simulink model "VD_correct"  (R2023b)
settings: Solver=ode113  StartTime=0.0  StopTime=20  MaxStep=0.4  RelTol=1e-3
libraries: simulink x2, slpidlib x1
settings Model: Creator=Supriya  LastModifiedBy=Supriya

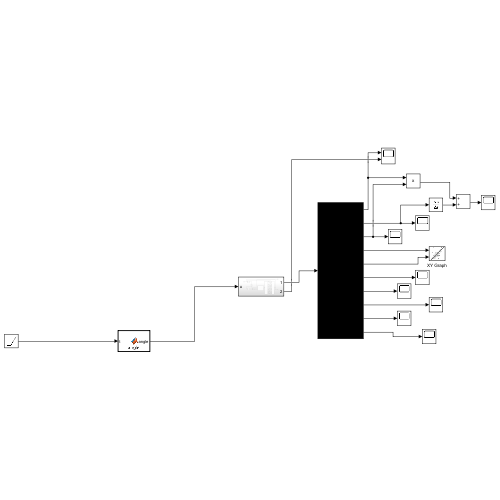
[thumbnail: Simulink's stored preview of the top-level diagram]
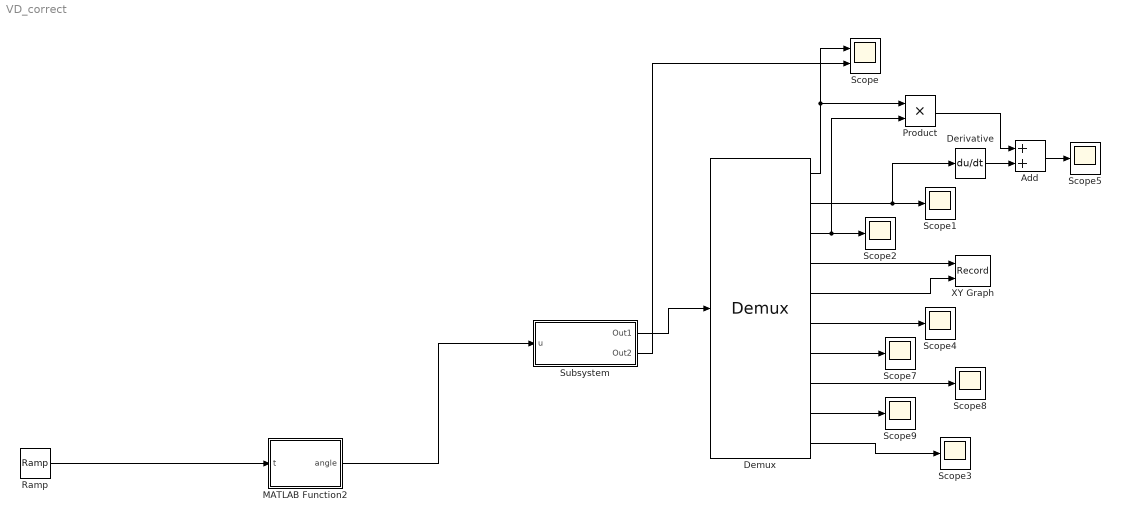
== system VD_correct ==
  Add : Sum
  Demux : Demux  Outputs=10
  Derivative : Derivative
  MATLAB Function2 : MATLAB Function  TreatAsAtomicUnit=on
  Product : Product
  Ramp : simulink/Sources/Ramp  slope=1  start=0  InitialOutput=0
  Scope : Scope  NumInputPorts=2
  Scope{1..5,7..9} (8 alike) : Scope
  Subsystem : Subsystem
  XY Graph : Record  FileSettingsInternal="{\"entries\":[{\"content\":{\"excelSettings\":{\"content\":{},\"type\":\"Streamout.ExcelSettings\"}},\"type\":\"Streamout.FileSettingStorage\",\"uuid\":\"\"}],\"packageUris\":[\"http:\\/\\/schema.mathworks.com\\/mf0\\/streamout_blocks\\/R2020a\"],\"version\":\"1.0\"}"  Layout=[1 1]  SignalsInternal="{\"entries\":[{\"content\":{\"signals\":[{\"content\":{\"blockPath\":[],\"dimensions\":[1],\"domain\":\"\",\"lineColor\":\"#a2142f\",\"plots\":[ 1 ],\"port\":1,\"sid\":[\"\"],\"signalID\":1,\"signalName\":\"Demux:4\"},\"type\":\"RecordBlkView.Signal\",\"uuid\":\"\"},{\"content\":{\"blockPath\":[],\"dimensions\":[1],\"domain\":\"\",\"lineColor\":\"#139fff\",\"plots\":[ 1 ],\"port\":2,\"sid\":[\"\"],\"signalID\":2,\"signalName\":\"Demux:5\"},\"type\":\"RecordBlkView.Signal\",\"uuid\":\"\"}]},\"type\":\"RecordBlkView.InputSignals\",\"uuid\":\"\"}],\"packageUris\":[\"http:\\/\\/schema.mathworks.com\\/mf0\\/streamout_blocks\\/R2020a\"],\"version\":\"1.0\"}"  VisualizationBindings="{\"xyplotplugin\":{\"info\":[{\"series\":[{\"bindingParametersList\":[{\"parameter\":\"X-Axis\",\"signalID\":1,\"signalName\":\"Demux:4\"},{\"parameter\":\"Y-Axis\",\"signalID\":2,\"signalName\":\"Demux:5\"}],\"seriesID\":0}],\"subplotID\":1}]}}"  CompatibilityTag=XY
  wires:
  Ramp/1 -> MATLAB Function2/1(t)
  MATLAB Function2/1(angle) -> Subsystem/1(u)
  Subsystem/1(Out1) -> Demux/1
  Demux/1 -> Scope/1, Product/1
  Demux/2 -> Derivative/1, Scope1/1
  Demux/3 -> Product/2, Scope2/1
  Demux/6 -> Scope4/1
  Demux/4 -> XY Graph/1
  Demux/5 -> XY Graph/2
  Demux/7 -> Scope7/1
  Demux/8 -> Scope8/1
  Demux/9 -> Scope9/1
  Demux/10 -> Scope3/1
  Product/1 -> Add/1
  Derivative/1 -> Add/2
  Add/1 -> Scope5/1
  Subsystem/2(Out2) -> Scope/2

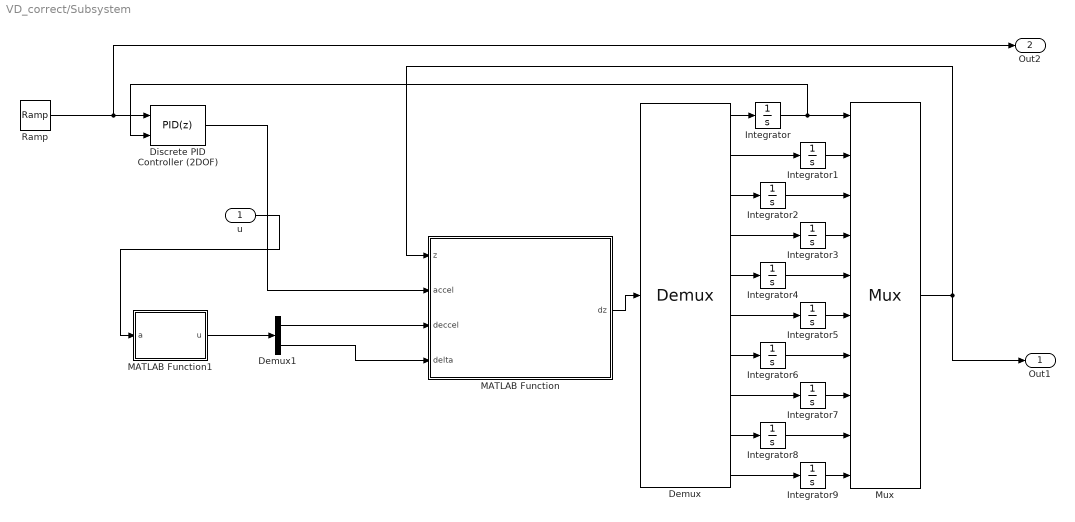
== system VD_correct/Subsystem ==
  u : Inport
  Demux : Demux  Outputs=10
  Demux1 : Demux  Outputs=2
  Discrete PID Controller (2DOF) : slpidlib/PID Controller (2DOF)  Controller=PID  Form=Parallel  TimeDomain=Discrete-time  UseExternalTs=off  SampleTime=-1  IntegratorMethod=Forward Euler  FilterMethod=Forward Euler  ControllerParametersSource=internal  P=6.4  I=8  UseKiTs=off  D=0.4  N=100  UseFilter=off  b=1  c=1  TunerSelectOption=Transfer Function Based (PID Tuner App)  InitialConditionSource=internal  InitialConditionForIntegrator=0  InitialConditionForFilter=0  DifferentiatorICPrevScaledInput=0  ExternalReset=none  TrackingMode=off  Kt=1  LimitOutput=off  SatLimitsSource=internal  UpperSaturationLimit=inf  LowerSaturationLimit=-inf  LinearizeAsGain=off  AntiWindupMode=none  Kb=1  LimitIntegrator=off  UpperIntegratorSaturationLimit=inf  LowerIntegratorSaturationLimit=-inf  POutMin=[]  POutMax=[]  IOutMin=[]  IOutMax=[]  DOutMin=[]  DOutMax=[]  NOutMin=[]  NOutMax=[]  bOutMin=[]  bOutMax=[]  cOutMin=[]  cOutMax=[]  SumOutMin=[]  SumOutMax=[]  SaturationOutMin=[]  SaturationOutMax=[]  PParamMin=[]  PParamMax=[]  IParamMin=[]  IParamMax=[]  DParamMin=[]  DParamMax=[]  NParamMin=[]  NParamMax=[]  bParamMin=[]  bParamMax=[]  cParamMin=[]  cParamMax=[]  KbParamMin=[]  KbParamMax=[]  KtParamMin=[]  KtParamMax=[]  KbOutMin=[]  KbOutMax=[]  KtOutMin=[]  KtOutMax=[]  IntegratorOutMin=[]  IntegratorOutMax=[]  FilterOutMin=[]  FilterOutMax=[]  SumI1OutMin=[]  SumI1OutMax=[]  SumI2OutMin=[]  SumI2OutMax=[]  SumI3OutMin=[]  SumI3OutMax=[]  SumI4OutMin=[]  SumI4OutMax=[]  SumDOutMin=[]  SumDOutMax=[]  Sum1OutMin=[]  Sum1OutMax=[]  Sum2OutMin=[]  Sum2OutMax=[]  Sum3OutMin=[]  Sum3OutMax=[]  DifferentiatorOutMin=[]  DifferentiatorOutMax=[]  FilterDiffOutCoefMin=[]  FilterDiffOutCoefMax=[]  ReciprocalOutMin=[]  ReciprocalOutMax=[]  SumDenOutMin=[]  SumDenOutMax=[]  SumNumOutMin=[]  SumNumOutMax=[]  DivideOutMin=[]  DivideOutMax=[]  UdiffTsProdOutMin=[]  UdiffTsProdOutMax=[]  NTsProdOutMin=[]  NTsProdOutMax=[]  UintegralTsProdOutMin=[]  UintegralTsProdOutMax=[]  UngainTsProdOutMin=[]  UngainTsProdOutMax=[]  ClampingZeroOutDataTypeStr=Inherit: Inherit via back propagation  ClampingZeroOutMin=[]  ClampingZeroOutMax=[]  FilterDenConstantOutDataTypeStr=Inherit: Inherit via back propagation  FilterDenConstantOutMin=[]  FilterDenConstantOutMax=[]  PCopyOutDataTypeStr=Inherit: Inherit via back propagation  PCopyOutMin=[]  PCopyOutMax=[]  NCopyOutDataTypeStr=Inherit: Inherit via back propagation  NCopyOutMin=[]  NCopyOutMax=[]  IntegratorContinuousStateAttributes=''  IntegratorStateMustResolveToSignalObject=off  IntegratorRTWStateStorageClass=Auto  FilterContinuousStateAttributes=''  FilterStateMustResolveToSignalObject=off  FilterRTWStateStorageClass=Auto  ParallelPVariant=InternalParameters  IdealPVariant=Disabled  IVariant=InternalParameters  DVariant=InternalParameters  bVariant=InternalParameters  cVariant=InternalParameters  IntegratorVariant=Discrete  SatVariant=Disabled  AWVariant=Passthrough  PCopyVariant=Disabled  TRVariant=Disabled  FdbkBlocksVariant=Forward  IdealPFdbkVariant=Disabled  SatFdbkVariant=Disabled  DerivativeFilterVariant=Differentiator  NVariant=Passthrough  NCopyVariant=Disabled_SignalSpec  FilterICVariant=InternalICsDifferentiator  IntegratorICVariant=InternalICs  ExternalResetVariant=Disabled  TRSumVariant=Passthrough  SumFdbkVariant=Disabled  SumVariant=Sum_PID  TsampFilterVariant=InternalTs  TsampNgainVariant=Passthrough  TsampIntegralVariant=Disabled_SignalSpec  ExternalSaturationOutDataTypeStr=Inherit: Same as second input
      settings: LibrarySourceBlock=simulink/Discrete/Discrete PID Controller (2DOF)
  Integrator : Integrator  InitialCondition=16
  Integrator{1..9} (9 alike) : Integrator
  MATLAB Function : MATLAB Function  TreatAsAtomicUnit=on
  MATLAB Function1 : MATLAB Function  TreatAsAtomicUnit=on
  Mux : Mux  Inputs=10
  Ramp : simulink/Sources/Ramp  slope=0.64  start=0  InitialOutput=16
  Out1 : Outport
  Out2 : Outport  Port=2
  wires:
  MATLAB Function/1(dz) -> Demux/1
  Demux/1 -> Integrator/1
  Integrator/1 -> Discrete PID Controller (2DOF)/2, Mux/1
  Demux/3 -> Integrator2/1
  Integrator2/1 -> Mux/3
  Integrator1/1 -> Mux/2
  Demux/2 -> Integrator1/1
  Demux/4 -> Integrator3/1
  Integrator3/1 -> Mux/4
  Integrator4/1 -> Mux/5
  Demux/5 -> Integrator4/1
  Demux/6 -> Integrator5/1
  Integrator5/1 -> Mux/6
  Demux/7 -> Integrator6/1
  Integrator6/1 -> Mux/7
  Demux/8 -> Integrator7/1
  Integrator7/1 -> Mux/8
  Demux/9 -> Integrator8/1
  Integrator8/1 -> Mux/9
  Demux/10 -> Integrator9/1
  Integrator9/1 -> Mux/10
  Mux/1 -> MATLAB Function/1(z), Out1/1
  u/1 -> MATLAB Function1/1(a)
  MATLAB Function1/1(u) -> Demux1/1
  Discrete PID Controller (2DOF)/1 -> MATLAB Function/2(accel)
  Ramp/1 -> Out2/1, Discrete PID Controller (2DOF)/1
  Demux1/1 -> MATLAB Function/3(deccel)
  Demux1/2 -> MATLAB Function/4(delta)

== matlab function VD_correct/Subsystem/MATLAB Function1 ==
  data: a input; u output
function u = u(a)
    u=[0, a];
end

== matlab function VD_correct/MATLAB Function2 ==
  data: t input; angle output
function angle = angle(t)
    % if t<1
    %     angle_steer = 0;%(pi/180) * sin(2*pi*0.1*t);
    % elseif 16>=t>=1
    %     angle_steer = 0.5*(pi/180)*t;
    % else
    %     angle_steer=8*(pi/180)*t;
    % end
    angle_steer = 3*(pi/180) * sin(2*pi*0.2*t);
    angle=angle_steer;
end

== matlab function VD_correct/Subsystem/MATLAB Function ==
  data: dz output; z input; accel input; deccel input; delta input
%This code is for state space of vehicle dynamics
% states: Vx, Vy, r

function dz = vehicle_dynamics(z, accel,deccel,delta)
    % abc = Forces
    % dt;
    %tic;    
    dz =zeros(10,1);
    params = system_parameters();
    Vx =  z(1);
    Vy = z(2);
    r  = z(3);
    x  = z(4);
    y  = z(5);
    psi= z(6);
    ax = -z(2) * r;
    ay = z(1) * r;

    %%input torue to each wheel 
    tau_in = cal_wheel_torque_in(params, accel, deccel);
    tau_in_fl = tau_in(1);
    tau_in_fr = tau_in(2);
    tau_in_rl = tau_in(3);
    tau_in_rr = tau_in(4);
    
    %% calculate forces
    t_forces = tire_forces(params, z, delta, ax, ay, deccel); %8 * 1 vector
    [Fx_sum, Fy_f, Fy_r, Fy_del] = vehicle_forces(params, z, t_forces, delta);
        
    Vx_dt = Vy * r + (Fx_sum / params.m);
    Vy_dt = -Vx * r + ((Fy_f+ Fy_r) / params.m);

    t_forces = tire_forces(params, z, delta, Vx_dt, Vy_dt,deccel); %8 * 1 vector
    [Fx_sum, Fy_f, Fy_r, Fy_del] = vehicle_forces(params, z, t_forces, delta);


    Vx_dt = Vy * r + (Fx_sum / params.m);
    Vy_dt = -Vx * r + ((Fy_f+ Fy_r) / params.m);
    r_dt =  (params.a * Fy_f - params.b *Fy_r + Fy_del) / params.Izz_v;

    x_dt = Vx * cos(psi) - Vy * sin(psi);
    y_dt = Vx * sin(psi) + Vy * cos(psi);
    psi_dt  = r;    

    %set tire forces 
    Fx_fl = t_forces(1);
    Fx_fr = t_forces(2);
    Fx_rl = t_forces(3);
    Fx_rr = t_forces(4); 

    %wheel velocities 
    w_fl_dt = (tau_in_fl - Fx_fl * params.R_f) / params.Iyy_w_f;
    w_fr_dt = (tau_in_fr - Fx_fr * params.R_f) / params.Iyy_w_f;
    w_rl_dt = (tau_in_rl - Fx_rl * params.R_r) / params.Iyy_w_r;
    w_rr_dt = (tau_in_rr - Fx_rr * params.R_r) / params.Iyy_w_r;

    omega_fl_dt = w_fl_dt;
    omega_fr_dt = w_fr_dt;
    omega_rl_dt = w_rl_dt;
    omega_rr_dt = w_rr_dt;
    %tp = toc;
    dz = [Vx_dt; Vy_dt; r_dt; x_dt; y_dt; psi_dt; omega_fl_dt; omega_fr_dt; omega_rl_dt; omega_rr_dt];

    % ax = (Vx_dt -ax)/dt;
    % ay = (Vy_dt - ay)/dt;
    % 
    %dz = [Vx_dt; Vy_dt; r_dt; x_dt; y_dt; psi_dt; omega_fl_dt; omega_fr_dt; omega_rl_dt; omega_rr_dt; ax; ay];
    function params = system_parameters();
        params.m = 2000; %kg
        params.rho = 1.225; %kg /m3
        params.C_d = 0.4; %
        params.Af = 1.6; %frontal area of vehicle 
        params.V_wind = 10 ;  %m/s
        params.a = 1.1;         %front_axel - CG
        params.b = 1.2;         % rear axel - CG
        params.l =  1.1 + 1.2;  %%m length of wheel base
        params.tf =  1.58; % track idth of wheel base 
        params.tr = 1.58; % track width of rear wheel base
        params.w = 1.58; % vehicle width
        params.Izz_v = 2000 * ((1.1+1.2)^2 + (1.58)^2) / 12;  %vehicle intertia 
        params.max_torque = 450; %Nm
        params.max_power =  225* 10^3;
        params.C_x = 50000 ;     %N
        params.C_y = 80000 ;  %N/Radlateral coefficient of stiffness
        params.R_f = 0.334; % m 
        params.R_r = 0.334; % m
        params.tire_m_f = 12; %mass in Kg
        params.tire_m_r = 12; %mass in Kg
        params.Iyy_w_f = 0.5 * 12 * 0.334; 
        params.Iyy_w_r = 0.5 * 12 * 0.334;
        % params.slip_max = (params.max_torque * accel / (params.R_f *2 * params.C_x));
        params.slip_min = -0.1;
        params.no_drive_wheels = 2;
        params.g = 9.8; %m/s2
        params.h = 0.25; %m
    end

end
